simulink model "lab2_EmulationSS_ContinuosTime_Nominal"  (R2020b)
settings: Solver=VariableStepAuto  StartTime=0.0  StopTime=10.0  RelTol=1e-3
undefined symbols (not defined in the file): A0, B0, C0, D0, K, Nu, Nx, sens, stepAmplitude
settings Model: Creator=Musta  LastModifiedBy=Musta

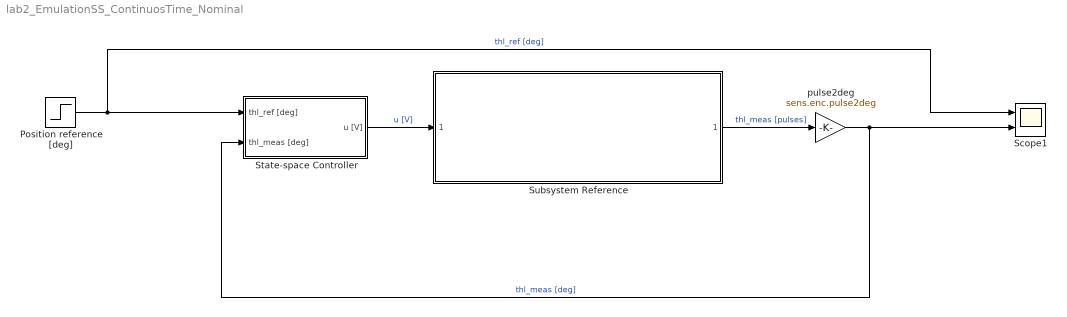
== system lab2_EmulationSS_ContinuosTime_Nominal ==
  Position reference [deg] : Step  Time=0  After=stepAmplitude  SampleTime=0
  Scope1 : Scope  NumInputPorts=2
  State-space Controller : Subsystem
  Subsystem Reference : Subsystem  ReferencedSubsystem=plant_model
  pulse2deg : Gain  Gain=sens.enc.pulse2deg
  wires:
  Position reference [deg]/1 -> Scope1/1, State-space Controller/1(thl_ref [deg])  "thl_ref [deg]"
  Subsystem Reference/1 -> pulse2deg/1  "thl_meas [pulses]"
  State-space Controller/1(u [V]) -> Subsystem Reference/1  "u [V]"
  pulse2deg/1 -> Scope1/2, State-space Controller/2(thl_meas [deg])  "thl_meas [deg]"

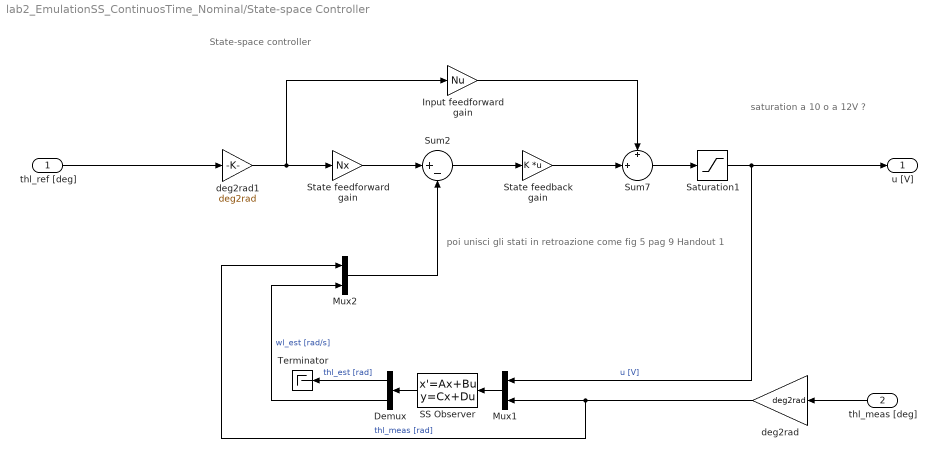
== system lab2_EmulationSS_ContinuosTime_Nominal/State-space Controller ==
  note: saturation a 10 o a 12V ?
  note: poi unisci gli stati in retroazione come fig 5 pag 9 Handout 1
  note: State-space controller
  thl_ref [deg] : Inport
  thl_meas [deg] : Inport  Port=2
  Demux : Demux  Outputs=2
  Input feedforward gain : Gain  Gain=Nu
  Mux1 : Mux  Inputs=2
  Mux2 : Mux  Inputs=2
  SS Observer : StateSpace  A=A0  B=B0  C=C0  D=D0  InitialCondition=0
  Saturation1 : Saturate  UpperLimit=12  LowerLimit=-12
  "State feedback gain " : Gain  Gain=K  Multiplication=Matrix(K*u) (u vector)
  State feedforward gain : Gain  Gain=Nx
  Sum2 : Sum  Inputs=|+-
  Sum7 : Sum  Inputs=+|+||
  Terminator : Terminator
  deg2rad : Gain  Gain=deg2rad
  deg2rad1 : Gain  Gain=deg2rad
  u [V] : Outport
  wires:
  "State feedback gain "/1 -> Sum7/2
  thl_meas [deg]/1 -> deg2rad/1
  deg2rad/1 -> Mux2/1, Mux1/2  "thl_meas [rad]"
  Sum7/1 -> Saturation1/1
  Input feedforward gain/1 -> Sum7/1
  deg2rad1/1 -> Input feedforward gain/1, State feedforward gain/1
  Saturation1/1 -> u [V]/1, Mux1/1  "u [V]"
  SS Observer/1 -> Demux/1
  Mux2/1 -> Sum2/2
  Mux1/1 -> SS Observer/1
  Sum2/1 -> "State feedback gain "/1
  State feedforward gain/1 -> Sum2/1
  thl_ref [deg]/1 -> deg2rad1/1
  Demux/2 -> Mux2/2  "wl_est [rad/s]"
  Demux/1 -> Terminator/1  "thl_est [rad]"
